simulink model "multi_input_isolated_boost_converter"  (R2020a)
settings: Solver=VariableStepAuto  StartTime=0.0  StopTime=1  RelTol=1e-3  EnableMultiTasking=on
libraries: powerlib x20, simulink x1, electricdrivelib x1
settings Model: Creator=sunil  LastModifiedBy=sunil
settings DataIOCC: ReturnWorkspaceOutputs=off
settings OptimizationCC: LifeSpan=inf
settings DebuggingCC: SFUnexpectedBacktrackingDiag=warning  SFNoUnconditionalDefaultTransitionDiag=warning  ArithmeticOperatorsInVariantConditions=warning
settings SFSimCC: SimUseLocalCustomCode=off  CustomCodeUndefinedFunction=UseInterfaceOnly
settings RTWCC: RTWUseLocalCustomCode=off
settings CodeAppCC: StateflowObjectComments=on
settings GRTTargetCC: TargetLangStandard=C89/C90 (ANSI)
settings ConfigComp: CovMetricSettings=dw  CovHtmlReporting=on  CovSaveCumulativeToWorkspaceVar=on  CovSaveSingleToWorkspaceVar=on  CovExternalEMLEnable=off
settings SimscapeCC: SimscapeNormalizeSystem=off

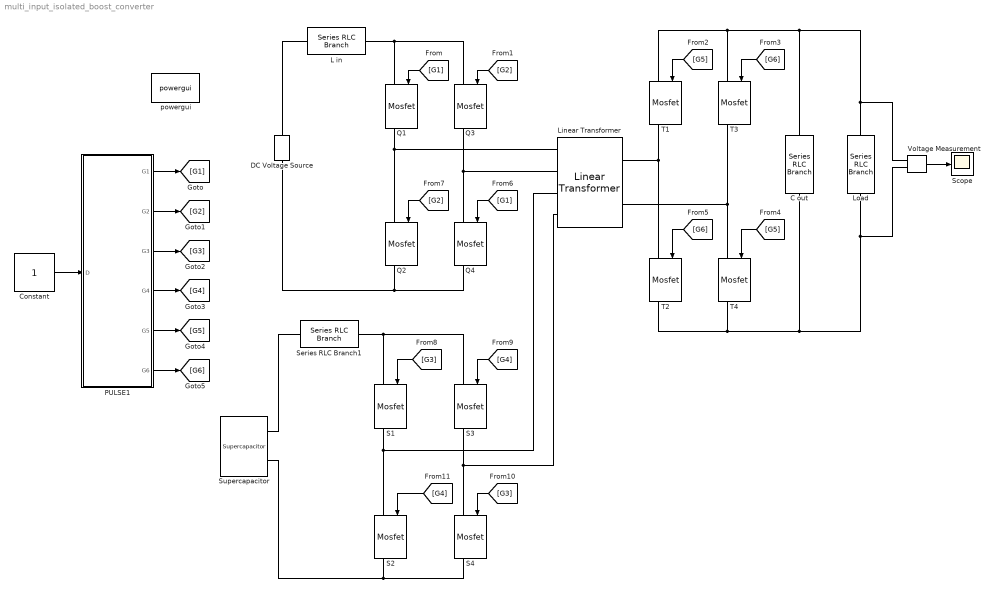
== system multi_input_isolated_boost_converter ==
  C out : powerlib/Elements/Series RLC Branch  LConnTagsString=__new0  RConnTagsString=__new0  BranchType=C  Resistance=1  Inductance=1e-3  SetiL0=off  InitialCurrent=0  Capacitance=150e-6  Setx0=off  InitialVoltage=0  Measurements=None
  Constant : Constant
  DC Voltage Source : powerlib/Electrical Sources/DC Voltage Source  Amplitude=288  Measurements=None
  L in : powerlib/Elements/Series RLC Branch  LConnTagsString=__new0  RConnTagsString=__new0  BranchType=L  Resistance=1  Inductance=175e-6  SetiL0=off  InitialCurrent=0  Capacitance=1e-6  Setx0=off  InitialVoltage=0  Measurements=None
  Linear Transformer : powerlib/Elements/Linear Transformer  UNITS=pu  NominalPower=[ 30000 50 ]  winding1="[576*1.414  0.002  0.015 ]"  winding2="[48*1.414  0.002  0.015 ]"  ThreeWindings=on  winding3=[288*1.414 0.002 0.015 ]  RmLm=[ 500 500 ]  Measurements=None  DataType=off
  Load : powerlib/Elements/Series RLC Branch  LConnTagsString=__new0  RConnTagsString=__new0  BranchType=R  Resistance=900  Inductance=1e-3  SetiL0=off  InitialCurrent=0  Capacitance=1e-6  Setx0=off  InitialVoltage=0  Measurements=None
  PULSE1 : Subsystem
  "Q1 " : powerlib/Power Electronics/Mosfet  Ron=0.1  Lon=0  Rd=0.01  Vfd=0  IC=0  Rs=1e5  Cs=inf  Measurements=on
  "Q2 " : powerlib/Power Electronics/Mosfet  Ron=0.1  Lon=0  Rd=0.01  Vfd=0  IC=0  Rs=1e5  Cs=inf  Measurements=on
  "Q3 " : powerlib/Power Electronics/Mosfet  Ron=0.1  Lon=0  Rd=0.01  Vfd=0  IC=0  Rs=1e5  Cs=inf  Measurements=on
  "Q4 " : powerlib/Power Electronics/Mosfet  Ron=0.1  Lon=0  Rd=0.01  Vfd=0  IC=0  Rs=1e5  Cs=inf  Measurements=on
  "S1 " : powerlib/Power Electronics/Mosfet  Ron=0.1  Lon=0  Rd=0.01  Vfd=0  IC=0  Rs=1e5  Cs=inf  Measurements=on
  "S2 " : powerlib/Power Electronics/Mosfet  Ron=0.1  Lon=0  Rd=0.01  Vfd=0  IC=0  Rs=1e5  Cs=inf  Measurements=on
  "S3 " : powerlib/Power Electronics/Mosfet  Ron=0.1  Lon=0  Rd=0.01  Vfd=0  IC=0  Rs=1e5  Cs=inf  Measurements=on
  "S4 " : powerlib/Power Electronics/Mosfet  Ron=0.1  Lon=0  Rd=0.01  Vfd=0  IC=0  Rs=1e5  Cs=inf  Measurements=on
  Scope : Scope
  Series RLC Branch1 : powerlib/Elements/Series RLC Branch  LConnTagsString=__new0  RConnTagsString=__new0  BranchType=L  Resistance=1  Inductance=175e-6  SetiL0=off  InitialCurrent=0  Capacitance=1e-6  Setx0=off  InitialVoltage=0  Measurements=None
  Supercapacitor : electricdrivelib/Extra Sources/Supercapacitor  C=99.5  Rdc=8.9e-3  Voltage=48  Ns=18  Np=1  Vinit=0  Temp=25  PresetModel=off  EstParam=off  Nc=1  r=1e-9  epsilon=6.0208e-10  Ich=10  Vstern="[0.161  2.7  7.8]"  Self_dis=on  Ioc=10  Vself="[48  47.8  47.06  44.65]"  demandeplot=off  I="[10  20 100  500]"  Units=sec  Vmax=0  If=0  deltaV=0  alpha=0  sec=0
      settings: SourceProductBaseCode=PS
  "T1 " : powerlib/Power Electronics/Mosfet  Ron=0.1  Lon=0  Rd=0.01  Vfd=0  IC=0  Rs=1e5  Cs=inf  Measurements=on
  "T2 " : powerlib/Power Electronics/Mosfet  Ron=0.1  Lon=0  Rd=0.01  Vfd=0  IC=0  Rs=1e5  Cs=inf  Measurements=on
  "T3 " : powerlib/Power Electronics/Mosfet  Ron=0.1  Lon=0  Rd=0.01  Vfd=0  IC=0  Rs=1e5  Cs=inf  Measurements=on
  "T4 " : powerlib/Power Electronics/Mosfet  Ron=0.1  Lon=0  Rd=0.01  Vfd=0  IC=0  Rs=1e5  Cs=inf  Measurements=on
  Voltage Measurement : powerlib/Measurements/Voltage Measurement  PhasorSimulation=off  OutputType=Complex  PSBequivalent=0
  powergui : powerlib/powergui  Priority=1  SimulationMode=Discrete  SampleTime=5e-6  frequency=60  Iterations=50  frequencyindice=0  Pbase=100e6  ErrMax=1e-4  UnitsV=kV  UnitsW=MW  buscounter=0  FunctionMessages=off  echomessages=off  EnableUseOfTLC=off  CurrentSourceSwitches=off  DisableSnubberDevices=off  DisableRonSwitches=off  DisableVfSwitches=off  DisplayEquations=off  AutomaticDiscreteSolvers=off  SolverType=Tustin/Backward Euler (TBE)  Interpol=off  ExternalGateDelay=off  methode=off  Ts=10  x0status=blocks  SPID=off  SwTol=0  HookPort=off  NonlinearTolerance=1e-4  nMaxIteration=100  ContinueOnMaxIteration=off  RestoreLinks=warning  ResistiveCurrentMeasurement=off  Frange=[0:2:500]  Ylog=off  Xlog=on  ShowGrid=off  save=off  variable=ZData  structure=0  ZoomFFT=off  StartTime=0.0  cycles=1  DisplayStyle=1  fundamental=60  FreqAxis=off  MaxFrequency=1000  frequencyindicesteady=1  RmsSteady=1  display=off
  wires:
  Voltage Measurement/1 -> Scope/1
  [G1] -> "Q1 "/1
  [G2] -> "Q3 "/1
  [G5] -> "T1 "/1
  [G6] -> "T3 "/1
  [G5] -> "T4 "/1
  [G1] -> "Q4 "/1
  [G2] -> "Q2 "/1
  [G3] -> "S1 "/1
  [G4] -> "S3 "/1
  [G3] -> "S4 "/1
  [G4] -> "S2 "/1
  [G6] -> "T2 "/1
  Constant/1 -> PULSE1/1(D)
  PULSE1/1(G1) -> [G1]
  PULSE1/2(G2) -> [G2]
  PULSE1/3(G3) -> [G3]
  PULSE1/4(G4) -> [G4]
  PULSE1/5(G5) -> [G5]
  PULSE1/6(G6) -> [G6]
  connections:
  DC Voltage Source/RConn1 -- L in/LConn1
  "Q3 "/RConn1 -- "Q4 "/LConn1 -- Linear Transformer/RConn3
  "Q2 "/LConn1 -- Linear Transformer/RConn4 -- "Q1 "/RConn1
  "Q1 "/LConn1 -- "Q3 "/LConn1 -- L in/RConn1
  "Q4 "/RConn1 -- "Q2 "/RConn1 -- DC Voltage Source/LConn1
  "S3 "/RConn1 -- "S4 "/LConn1 -- Linear Transformer/RConn1
  "S1 "/RConn1 -- Linear Transformer/RConn2 -- "S2 "/LConn1
  Series RLC Branch1/RConn1 -- "S3 "/LConn1 -- "S1 "/LConn1
  "S4 "/RConn1 -- Supercapacitor/LConn2 -- "S2 "/RConn1
  Supercapacitor/LConn1 -- Series RLC Branch1/LConn1
  "T3 "/RConn1 -- Linear Transformer/LConn1 -- "T4 "/LConn1
  "T2 "/LConn1 -- "T1 "/RConn1 -- Linear Transformer/LConn2
  "T1 "/LConn1 -- "T3 "/LConn1 -- C out/LConn1 -- Load/LConn1 -- Voltage Measurement/LConn1
  "T4 "/RConn1 -- C out/RConn1 -- Load/RConn1 -- Voltage Measurement/LConn2 -- "T2 "/RConn1

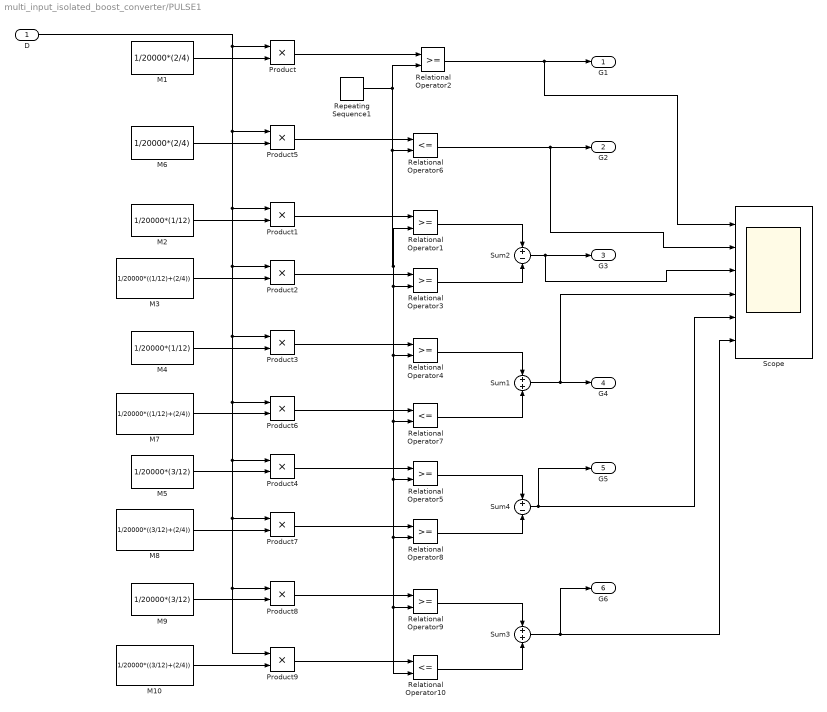
== system multi_input_isolated_boost_converter/PULSE1 ==
  D : Inport
  M1 : Constant  Value=1/20000*(2/4)
  M10 : Constant  Value=1/20000*((3/12)+(2/4))
  M2 : Constant  Value=1/20000*(1/12)
  M3 : Constant  Value=1/20000*((1/12)+(2/4))
  M4 : Constant  Value=1/20000*(1/12)
  M5 : Constant  Value=1/20000*(3/12)
  M6 : Constant  Value=1/20000*(2/4)
  M7 : Constant  Value=1/20000*((1/12)+(2/4))
  M8 : Constant  Value=1/20000*((3/12)+(2/4))
  M9 : Constant  Value=1/20000*(3/12)
  Product{,1..9} (10 alike) : Product
  Relational Operator{1..5,8..9} (7 alike) : RelationalOperator  OutDataTypeStr=boolean  RndMeth=Nearest
  Relational Operator10 : RelationalOperator  Operator=<=  OutDataTypeStr=boolean  RndMeth=Nearest
  Relational Operator6 : RelationalOperator  Operator=<=  OutDataTypeStr=boolean  RndMeth=Nearest
  Relational Operator7 : RelationalOperator  Operator=<=  OutDataTypeStr=boolean  RndMeth=Nearest
  Repeating Sequence1 : simulink/Sources/Repeating Sequence  rep_seq_t=[0 1/20000]  rep_seq_y=[0 1/20000]
  Scope : Scope  NumInputPorts=6
  Sum1 : Sum
  Sum2 : Sum  Inputs=+-
  Sum3 : Sum
  Sum4 : Sum  Inputs=+-
  G1 : Outport
  G2 : Outport  Port=2
  G3 : Outport  Port=3
  G4 : Outport  Port=4
  G5 : Outport  Port=5
  G6 : Outport  Port=6
  wires:
  Relational Operator2/1 -> Scope/1, G1/1
  Relational Operator6/1 -> Scope/2, G2/1
  M1/1 -> Product/2
  Product/1 -> Relational Operator2/1
  Product5/1 -> Relational Operator6/1
  M6/1 -> Product5/2
  Sum2/1 -> Scope/3, G3/1
  Relational Operator1/1 -> Sum2/1
  Sum1/1 -> Scope/4, G4/1
  M2/1 -> Product1/2
  M3/1 -> Product2/2
  M4/1 -> Product3/2
  Product1/1 -> Relational Operator1/1
  Product2/1 -> Relational Operator3/1
  Product3/1 -> Relational Operator4/1
  Relational Operator3/1 -> Sum2/2
  Relational Operator4/1 -> Sum1/1
  Product6/1 -> Relational Operator7/1
  M7/1 -> Product6/2
  Relational Operator7/1 -> Sum1/2
  Repeating Sequence1/1 -> Relational Operator2/2, Relational Operator10/2, Relational Operator9/2, Relational Operator8/2, Relational Operator5/2, Relational Operator7/2, Relational Operator4/2, Relational Operator3/2, Relational Operator1/2, Relational Operator6/2
  D/1 -> Product9/1, Product8/1, Product7/1, Product4/1, Product6/1, Product3/1, Product2/1, Product1/1, Product5/1, Product/1
  Sum4/1 -> G5/1, Scope/5
  Relational Operator5/1 -> Sum4/1
  Sum3/1 -> G6/1, Scope/6
  M5/1 -> Product4/2
  M8/1 -> Product7/2
  M9/1 -> Product8/2
  Product4/1 -> Relational Operator5/1
  Product7/1 -> Relational Operator8/1
  Product8/1 -> Relational Operator9/1
  Relational Operator8/1 -> Sum4/2
  Relational Operator9/1 -> Sum3/1
  Product9/1 -> Relational Operator10/1
  M10/1 -> Product9/2
  Relational Operator10/1 -> Sum3/2
